simulink model "hev_simulation"  (R2016b)
settings: Solver=FixedStepAuto  StartTime=0  StopTime=100  FixedStep=0.100000  RelTol=1e-3
values from neighbouring files (symbols this model uses):
  eta_Pe = eta_conv*eta_gen    (= 0.855)    [hev_parameters.m]
  eta_Pout = eta_inv*eta_im*eta_gear    (= 0.8379)    [hev_parameters.m]
  Fstart = m*3*9.8/1000    (= 1507.6908)    [hev_engine.m]    (also in hev_parameters.m)
  Ft_max = zeros(1,101)    [hev_parameters.m]
  Ft_min = zeros(1,101)    [hev_parameters.m]
  m = (mv+mp)*iv    (= 51282)    [hev_engine.m]    (also in hev_parameters.m)
  maxacc = 2.3/3.6    (= 0.638888888889)    [hev_parameters.m]
  maxdec = -2.0/3.6    (= -0.555555555556)    [hev_parameters.m]
  notch_ref = [repmat(1,1,40) repmat(0,1,20) repmat(-1,1,20) repmat(0,1,100)]    [hev_drivecycle.m]
  Paux = 30000    [hev_parameters.m]
  Pes_low = 200000    [hev_parameters.m]
  Pes_max = 330000    [hev_parameters.m]
  Pes_off = 0    [hev_parameters.m]
  Pes_opt = 280000    [hev_parameters.m]
  Q0 = 22    [hev_parameters.m]
  r0 = 554.9    [hev_parameters.m]
  r1 = 20.3    [hev_parameters.m]
  r2 = 3.56    [hev_parameters.m]
  Ri = 0.1    [hev_parameters.m]
  TPe = 0.2    [hev_parameters.m]
  Uoc = 692    [hev_parameters.m]
  v_ref = zeros(1,length(notch_ref))    [hev_drivecycle.m]
undefined symbols (not defined in the file or in its folder): MPCController
settings Model: Creator=Niklas  LastModifiedBy=Niklas
settings DataIOCC: SaveOutput=off  SignalLogging=off  DSMLogging=off

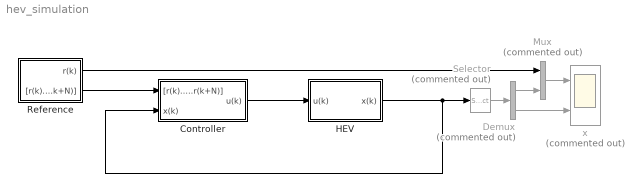
== system hev_simulation ==
  Controller : Subsystem
  Demux : Demux  Commented=on  Outputs=2
  HEV : Subsystem
  Mux : Mux  Commented=on  Inputs=2
  Reference : Subsystem
  Selector : Selector  Commented=on  InputPortWidth=3  IndexOptions=Index vector (dialog)  Indices=[2 3]  OutputSizes=1
  x : Scope  Commented=on  NumInputPorts=2
  wires:
  HEV/1(x(k)) -> Selector/1, Controller/2(x(k))
  Mux/1 -> x/1
  Reference/2("[r(k)...r(k+N)]") -> Controller/1("[r(k)...r(k+N)]")
  Reference/1(r(k)) -> Mux/1
  Selector/1 -> Demux/1
  Demux/1 -> Mux/2
  Demux/2 -> x/2
  Controller/1(u(k)) -> HEV/1(u(k))

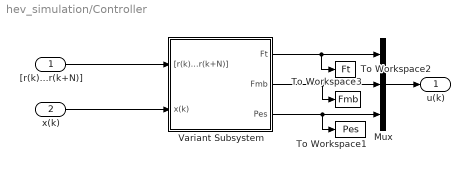
== system hev_simulation/Controller ==
  "[r(k)...r(k+N)]" : Inport
  x(k) : Inport  Port=2
  Mux : Mux  Inputs=3
  To Workspace1 : ToWorkspace  VariableName=Pes  SaveFormat=Structure  SampleTime=-1
  To Workspace2 : ToWorkspace  VariableName=Ft  SaveFormat=Structure  SampleTime=-1
  To Workspace3 : ToWorkspace  VariableName=Fmb  SaveFormat=Structure  SampleTime=-1
  Variant Subsystem : Subsystem  Variant=on
  u(k) : Outport
  wires:
  Mux/1 -> u(k)/1
  "[r(k)...r(k+N)]"/1 -> Variant Subsystem/1("[r(k)...r(k+N)]")
  x(k)/1 -> Variant Subsystem/2(x(k))
  Variant Subsystem/3(Pes) -> To Workspace1/1, Mux/3
  Variant Subsystem/2(Fmb) -> To Workspace3/1, Mux/2
  Variant Subsystem/1(Ft) -> Mux/1, To Workspace2/1

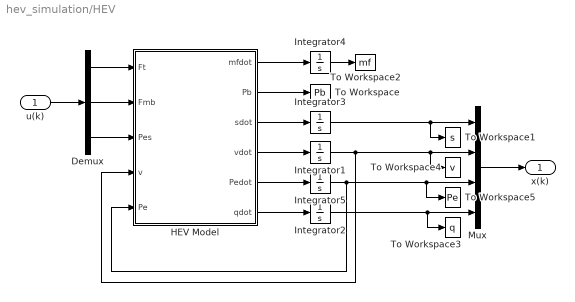
== system hev_simulation/HEV ==
  u(k) : Inport
  Demux : Demux  Outputs=3
  HEV Model : MATLAB Function  TreatAsAtomicUnit=on
  Integrator1 : Integrator  LowerSaturationLimit=0  ContinuousStateAttributes='v'
  Integrator2 : Integrator  InitialCondition=0.55  LimitOutput=on  UpperSaturationLimit=1  LowerSaturationLimit=0  ContinuousStateAttributes='q'
  Integrator3 : Integrator  LowerSaturationLimit=0  ContinuousStateAttributes='s'
  Integrator4 : Integrator  LowerSaturationLimit=0  ContinuousStateAttributes='v'
  Integrator5 : Integrator  UpperSaturationLimit=330000  LowerSaturationLimit=0  ContinuousStateAttributes='Pe'
  Mux : Mux
  To Workspace : ToWorkspace  VariableName=Pb  SaveFormat=Structure  SampleTime=-1
      settings: Save2DSignal=2-D array (concatenate along first dimension)
  To Workspace1 : ToWorkspace  VariableName=s  SaveFormat=Structure  SampleTime=-1
      settings: Save2DSignal=2-D array (concatenate along first dimension)
  To Workspace2 : ToWorkspace  VariableName=mf  SaveFormat=Structure  SampleTime=-1
      settings: Save2DSignal=2-D array (concatenate along first dimension)
  To Workspace3 : ToWorkspace  VariableName=q  SaveFormat=Structure  SampleTime=-1
  To Workspace4 : ToWorkspace  VariableName=v  SaveFormat=Structure  SampleTime=-1
  To Workspace5 : ToWorkspace  VariableName=Pe  SaveFormat=Structure  SampleTime=-1
  x(k) : Outport
  wires:
  u(k)/1 -> Demux/1
  Demux/2 -> HEV Model/2(Fmb)
  Demux/1 -> HEV Model/1(Ft)
  HEV Model/4(vdot) -> Integrator1/1
  HEV Model/6(qdot) -> Integrator2/1
  Integrator1/1 -> HEV Model/4(v), To Workspace4/1, Mux/2
  Mux/1 -> x(k)/1
  HEV Model/2(Pb) -> To Workspace/1
  Integrator2/1 -> Mux/4, To Workspace3/1
  HEV Model/3(sdot) -> Integrator3/1
  Integrator3/1 -> To Workspace1/1, Mux/1
  HEV Model/1(mfdot) -> Integrator4/1
  Integrator4/1 -> To Workspace2/1
  HEV Model/5(Pedot) -> Integrator5/1
  Integrator5/1 -> To Workspace5/1, Mux/3, HEV Model/5(Pe)
  Demux/3 -> HEV Model/3(Pes)

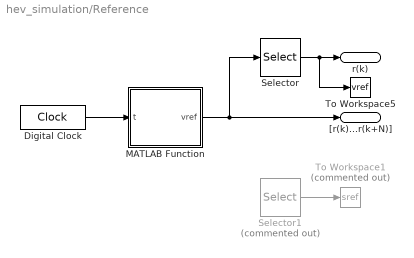
== system hev_simulation/Reference ==
  Digital Clock : DigitalClock
  MATLAB Function : MATLAB Function  TreatAsAtomicUnit=on
  Selector : Selector  InputPortWidth=41  IndexOptions=Starting index (dialog)  Indices=[1]  OutputSizes=1
  Selector1 : Selector  Commented=on  InputPortWidth=41  IndexOptions=Starting index (dialog)  Indices=[1]  OutputSizes=1
  To Workspace1 : ToWorkspace  Commented=on  VariableName=sref  SaveFormat=Structure  SampleTime=-1
      settings: Save2DSignal=2-D array (concatenate along first dimension)
  To Workspace5 : ToWorkspace  VariableName=vref  SaveFormat=Structure  SampleTime=0.1
      settings: Save2DSignal=2-D array (concatenate along first dimension)
  r(k) : Outport
  "[r(k)...r(k+N)]" : Outport  Port=2
  wires:
  Digital Clock/1 -> MATLAB Function/1(t)
  Selector/1 -> r(k)/1, To Workspace5/1
  MATLAB Function/1(vref) -> Selector/1, "[r(k)...r(k+N)]"/1
  Selector1/1 -> To Workspace1/1

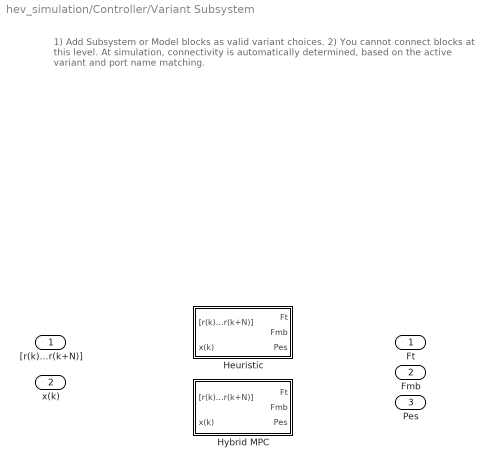
== system hev_simulation/Controller/Variant Subsystem ==
  note: 1) Add Subsystem or Model blocks as valid variant choices.
      | 2) You cannot connect blocks at this level. At simulation, connectivity is automatically
      | determined, based on the active variant and port name matching.
  "[r(k)...r(k+N)]" : Inport
  x(k) : Inport  Port=2
  Heuristic : Subsystem  VariantControl=controller == 1
  Hybrid MPC : Subsystem  VariantControl=controller == 2
  Ft : Outport
  Fmb : Outport  Port=2
  Pes : Outport  Port=3

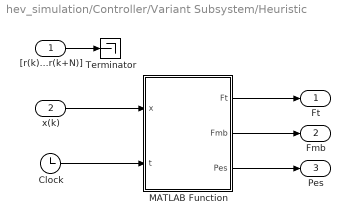
== system hev_simulation/Controller/Variant Subsystem/Heuristic ==
  "[r(k)...r(k+N)]" : Inport
  x(k) : Inport  Port=2  PortDimensions=4
  Clock : Clock
  MATLAB Function : MATLAB Function  TreatAsAtomicUnit=on
  Terminator : Terminator
  Ft : Outport
  Fmb : Outport  Port=2
  Pes : Outport  Port=3
  wires:
  MATLAB Function/1(Ft) -> Ft/1
  MATLAB Function/2(Fmb) -> Fmb/1
  x(k)/1 -> MATLAB Function/1(x)
  Clock/1 -> MATLAB Function/2(t)
  "[r(k)...r(k+N)]"/1 -> Terminator/1
  MATLAB Function/3(Pes) -> Pes/1

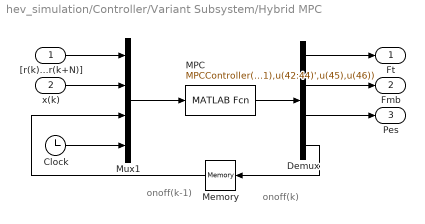
== system hev_simulation/Controller/Variant Subsystem/Hybrid MPC ==
  note: onoff(k)
  note: onoff(k-1)
  "[r(k)...r(k+N)]" : Inport
  x(k) : Inport  Port=2
  Clock : Clock
  Demux : Demux
  MPC : MATLABFcn  MATLABFcn=MPCController(u(1:41),u(42:44)',u(45),u(46))  OutputDimensions=3
  Memory : Memory  X0=1
  Mux1 : Mux
  Ft : Outport
  Fmb : Outport  Port=2
  Pes : Outport  Port=3
  wires:
  Mux1/1 -> MPC/1
  Clock/1 -> Mux1/4
  MPC/1 -> Demux/1
  Memory/1 -> Mux1/3
  Demux/1 -> Ft/1
  x(k)/1 -> Mux1/2
  "[r(k)...r(k+N)]"/1 -> Mux1/1
  Demux/4 -> Memory/1
  Demux/2 -> Fmb/1
  Demux/3 -> Pes/1

== matlab function hev_simulation/Reference/MATLAB Function ==
  data: t input; v_ref parameter; vref output
function vref  = fcn(t,v_ref)
N=41;
vref = v_ref(t+1:t+N);

== matlab function hev_simulation/HEV/HEV Model ==
  data: mfdot output; Pb output; sdot output; Ft input; Fmb input; Pes input; v input; Pe input; vdot output; Pedot output; qdot output; eta_Pe parameter; eta_Pout parameter; Paux parameter; m parameter; r0 parameter; r1 parameter; r2 parameter; TPe parameter; Q0 parameter; Ri parameter; Uoc parameter
function [mfdot,Pb,sdot,vdot,Pedot,qdot] = fcn(Ft, Fmb, Pes, v, Pe, eta_Pe, eta_Pout, Paux, m, r0, r1, r2, TPe, Q0, Ri, Uoc)

% Fuel consumption
if round(Pes) == 0
    mfdot = 0;
else
    kPes = Pes/1000;
    mfdot = (0.00413*kPes^2 - 2.22089*kPes + 499.19)*(1/3600)*kPes;
end

% Battery power
Pb = eta_Pout*Ft*v - eta_Pe*Pe + Paux;

% xdot = f(x,u)
sdot = v;
vdot = Ft/m - Fmb/m - (r2*v^2 + r1*v + r0)/m;
Pedot = (Pes - Pe)/TPe;
qdot = -(Uoc - sqrt(Uoc^2 - 4*Pb*Ri))/(2*3600*Q0*Ri);

== matlab function hev_simulation/Controller/Variant Subsystem/Heuristic/MATLAB Function ==
  data: x input; t input; v_ref parameter; notch_ref parameter; m parameter; maxacc parameter; maxdec parameter; Fstart parameter; Ft_max parameter; Ft_min parameter; Ft output; Fmb output; Pes_max parameter; Pes_opt parameter; Pes_low parameter; Pes_off parameter; Pes output
function [Ft, Fmb, Pes] = fcn(x, t, v_ref, notch_ref, m, maxacc, maxdec, Fstart, Ft_max, Ft_min, Pes_max, Pes_opt, Pes_low, Pes_off)

t = floor(t);
v = x(2)*3.6;
q = x(4);

% Determine Ft & Fmb
switch notch_ref(t+1)
    case 1
        % Ftmax
        if v <= 20
            Ft = m*maxacc + Fstart;
        elseif v <= 70
            Ft = Ft_max(21)*(20/v);
        else
            Ft = Ft_max(21)*(20/v)*(70/v);
        end
        Fmb = 0;
    case 0
        Ft = 0;
        Fmb = 0;
    case -1
        %Ftmin
        if v <= 42
            Ft = m*maxdec;
        else
            Ft = m*maxdec*(42/v);
        end
        Fmb = Ft - Ft_min(1);
    otherwise
        error('Invalid notch_ref!');
end

% Determine Pes
% Mode A
if v <= 25 && q >= 0.5
    switch notch_ref(t+1)
        case 1
            Pes = Pes_off;
        case 0
            Pes = Pes_off;
        case -1
            Pes = Pes_off;
        otherwise
            error('Invalid runmode!');
    end
% Mode E
elseif v <= 25 && q <= 0.5
    switch notch_ref(t+1)
        case 1
            Pes = Pes_max;
        case 0
            Pes = Pes_max;
        case -1
            Pes = Pes_low;
        otherwise
            error('Invalid runmode!');    
    end
% Mode B
elseif v >= 25 && q >= 0.25 && q <= 0.75
    switch notch_ref(t+1)
        case 1
            Pes = Pes_opt;
        case 0
            Pes = Pes_low;
        case -1
            Pes = Pes_off;
        otherwise
            error('Invalid runmode!');    
    end
% Mode C
elseif v >= 25 && q >= 0.2 && q <= 0.25
    switch notch_ref(t+1)
        case 1
            Pes = Pes_max;
        case 0
            Pes = Pes_max;
        case -1
            Pes = Pes_low;
        otherwise
            error('Invalid runmode!');    
    end
% Mode D
elseif v >= 25 && q >= 0.75 && q <= 0.8
    switch notch_ref(t+1)
        case 1
            Pes = Pes_off;
        case 0
            Pes = Pes_off;
        case -1
            Pes = Pes_off;
        otherwise
            error('Invalid runmode!');    
    end
else
    error('No mode satisfied');
end
